simulink model "DSB_TC_Receiver_Part_2_1"  (R2022a)
settings: Solver=FixedStepDiscrete  StartTime=0.0  StopTime=inf  RelTol=1e-3
PreLoadFcn:
  | addpath('matlab/DSB_TC');
libraries: dspsnks4 x1, dsparch4 x1, dspvision x1, dspstat3 x1, dspsigops x1, matrix_library x1
settings Model: Creator=vovan  LastModifiedBy=vovan

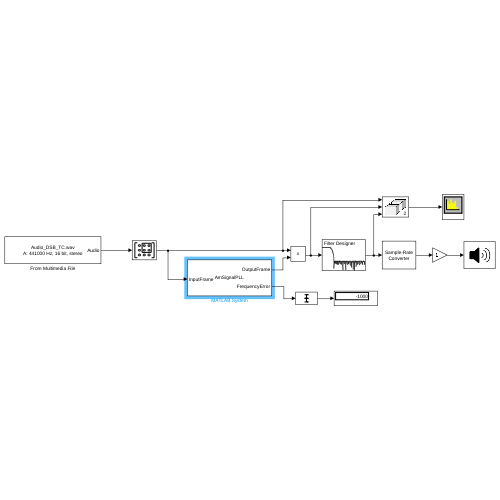
[thumbnail: Simulink's stored preview of the top-level diagram]
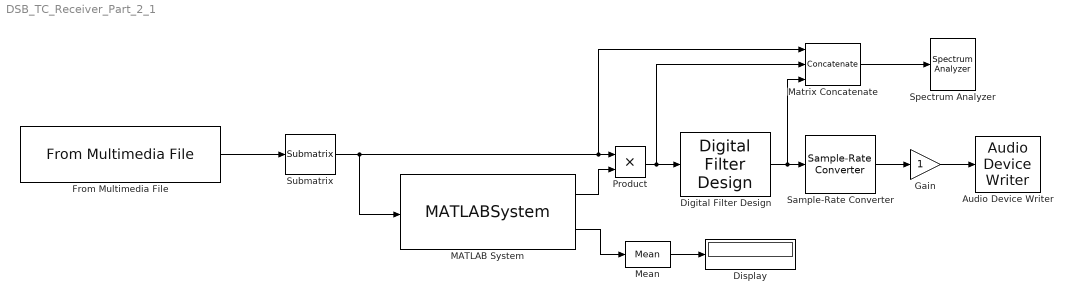
== system DSB_TC_Receiver_Part_2_1 ==
  Audio Device Writer : dspsnks4/Audio Device Writer  Driver=ALSA  Device=Default  InheritSampleRate=on  SampleRate=44100  BitDepth=16-bit integer  BufferSize=4096  NumBuffers=10  DefaultOutputChannelMapping=on  OutputChannelMapping=1:2  OutputNumUnderrunSamples=off  DriverIdx=8  DeviceWarnFlag=''
  Digital Filter Design : dsparch4/Digital Filter Design  mwdsp_browser_bugfix_var=off
  Display : Display
  From Multimedia File : dspvision/From Multimedia File  inputFilename=wav/Audio_DSB_TC.wav  readRange=[1 Inf]  loop=on  numPlays=inf  outputStreams=Audio only  videoDataType=single  audioDataType=double  inheritSampleTime=on  userDefinedSampleTime=1/30  noAudioOutput=off  isIntensityVideo=off  fourcc=RGB  colorVideoFormat=Separate color signals  outputEOF=off  dataOrg=Column-major  audioFrameSize=10000  computeAudioFrameSize=off  outSamplingMode=Sample based
  Gain : Gain
  MATLAB System : MATLABSystem  System=AmSignalPLL  SampleFrequency=441000  NoiseBandwidth=300  Dampingfactor=0.7  CentralFrequency=60e3 + 1000  SignalAmp=0.27  SimulateUsing=Code generation
      mask Type: AmSignalPLL
      mask Display:
      | disp('AmSignalPLL');
      | port_label('input',1,'InputFrame');
      | port_label('output',1,'OutputFrame');
      | port_label('output',2,'FrequencyError');
  Matrix Concatenate : Concatenate  NumInputs=3  Mode=Multidimensional array  ConcatenateDimension=2
  Mean : dspstat3/Mean  run=off  InputProcessing=Columns as channels (frame based)  reset_popup=None  directionMode=Each column  dimension=1  roiEnable=off  roiType=Rectangles  roiPortion=Entire ROI  roiOutput=Individual statistics for each ROI  roiFlag=off  roundingMode=Floor  overflowMode=off  outputDataTypeStr=Inherit: Same as accumulator  outputMin=[]  outputMax=[]  outputLastDataTypeStr=Inherit: Same as accumulator
  Product : Product
  Sample-Rate Converter : dspsigops/Sample-Rate Converter  InputSampleRate=441000  OutputSampleRate=44100  OutputRateTolerance=0  Bandwidth=40e3  StopbandAttenuation=80  SimulateUsing=Code generation
      settings: SourceProductBaseCode=DS
  Spectrum Analyzer : SpectrumAnalyzer
  Submatrix : matrix_library/Submatrix  RowSpan=All rows  RowStartMode=First  RowStartIndex=1  RowEndMode=Last  RowEndIndex=1  ColSpan=Range of columns  ColStartMode=First  ColStartIndex=1  ColEndMode=Index  ColEndIndex=1
      settings: SourceProductBaseCode=SL
  wires:
  From Multimedia File/1 -> Submatrix/1
  Submatrix/1 -> MATLAB System/1, Matrix Concatenate/1, Product/1
  MATLAB System/1 -> Product/2
  Product/1 -> Matrix Concatenate/2, Digital Filter Design/1
  Digital Filter Design/1 -> Matrix Concatenate/3, Sample-Rate Converter/1
  Sample-Rate Converter/1 -> Gain/1
  Gain/1 -> Audio Device Writer/1
  Matrix Concatenate/1 -> Spectrum Analyzer/1
  MATLAB System/2 -> Mean/1
  Mean/1 -> Display/1
